simulink model "AutomaticParking_Parallel_UtilityTruck"  (Simulink 10.2)
settings: Solver=ode45  StartTime=0  StopTime=60  FixedStep=0.002  RelTol=1e-3  AbsTol=1e-6
libraries: robotlib x11, Solver_SF x1, simulink x1
(part 1 of 3)
settings Model: Creator=pmather  LastModifiedBy=DwigHT  ExtModeTrigMode=oneshot  ExtModeArmWhenConnect=off
settings OptimizationCC: BlockReduction=off  BooleanDataType=off  InitFltsAndDblsToZero=on  LifeSpan=auto
settings DebuggingCC: SaveWithParameterizedLinksMsg=none  SignalResolutionControl=TryResolveAllWithWarning  MultiTaskDSMMsg=warning  MultiTaskCondExecSysMsg=none  FcnCallInpInsideContextMsg=error  SFUnexpectedBacktrackingDiag=error  SFNoUnconditionalDefaultTransitionDiag=error  SFExecutionAtInitializationDiag=warning
settings HardwareCC: TargetUnknown=on
settings SFSimCC: SimUseLocalCustomCode=on
settings RTWCC: TemplateMakefile=grt_vc.tmf  RTWUseLocalCustomCode=on
settings CodeAppCC: StateflowObjectComments=off
settings ConfigComp: CovExternalEMLEnable=on

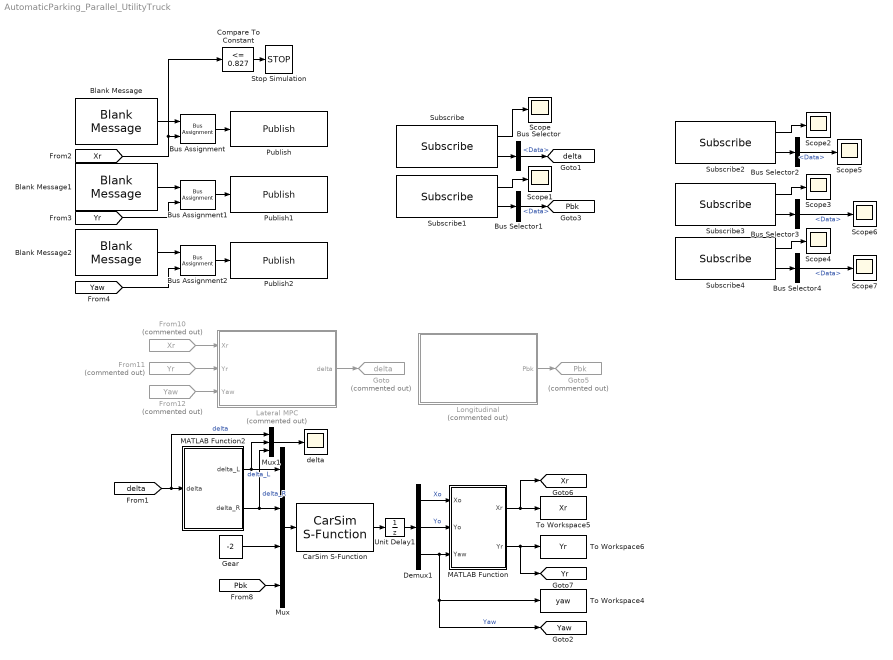
== system AutomaticParking_Parallel_UtilityTruck ==
  Blank Message : robotlib/Blank Message  messageClass=Message  entityType=std_msgs/Float64  messageType=std_msgs/Float64  SampleTime=inf  legacyBusStruct=off
  Blank Message1 : robotlib/Blank Message  messageClass=Message  entityType=std_msgs/Float64  messageType=std_msgs/Float64  SampleTime=inf  legacyBusStruct=off
  Blank Message2 : robotlib/Blank Message  messageClass=Message  entityType=std_msgs/Float64  messageType=std_msgs/Float64  SampleTime=inf  legacyBusStruct=off
  Bus Assignment : BusAssignment  AssignedSignals=Data
  Bus Assignment1 : BusAssignment  AssignedSignals=Data
  Bus Assignment2 : BusAssignment  AssignedSignals=Data
  Bus Selector{,1..4} (5 alike) : BusSelector  OutputSignals=Data
  CarSim S-Function : Solver_SF/CarSim S-Function  Priority=1  VehicleCode=i_s  SIMFILE=simfile
  Compare To Constant : simulink/Logic and Bit Operations/Compare To Constant  relop=<=  const=0.827  OutDataTypeStr=boolean
  Demux1 : Demux  Outputs=3
  From10 : From  Commented=on  GotoTag=Xr  TagVisibility=global
  From11 : From  Commented=on  GotoTag=Yr  TagVisibility=global
  From12 : From  Commented=on  GotoTag=Yaw  TagVisibility=global
  Gear : Constant  Value=-2
  Goto : Goto  Commented=on  GotoTag=delta  TagVisibility=global
  Goto5 : Goto  Commented=on  GotoTag=Pbk  TagVisibility=global
  Lateral MPC : Subsystem  Commented=on
  Longitudinal : Subsystem  Commented=on
  MATLAB Function : MATLAB Function  TreatAsAtomicUnit=on
  MATLAB Function2 : MATLAB Function  TreatAsAtomicUnit=on
  Mux : Mux
  Mux1 : Mux  Inputs=3
  Publish : robotlib/Publish  topicSource=Specify your own  topic=/Xr  messageType=std_msgs/Float64  legacyBusStruct=off  messageQueueLength=1
  Publish1 : robotlib/Publish  topicSource=Specify your own  topic=/Yr  messageType=std_msgs/Float64  legacyBusStruct=off  messageQueueLength=1
  Publish2 : robotlib/Publish  topicSource=Specify your own  topic=/Yaw  messageType=std_msgs/Float64  legacyBusStruct=off  messageQueueLength=1
  Scope{,1..7} (8 alike) : Scope
  Stop Simulation : Stop
  Subscribe : robotlib/Subscribe  topicSource=Specify your own  topic=/delta  messageType=std_msgs/Float64  SampleTime=-1  legacyBusStruct=off  messageQueueLength=1
  Subscribe1 : robotlib/Subscribe  topicSource=Specify your own  topic=/Pbk  messageType=std_msgs/Float64  SampleTime=-1  legacyBusStruct=off  messageQueueLength=1
  Subscribe2 : robotlib/Subscribe  topicSource=Specify your own  topic=/delta_t  messageType=std_msgs/Float64  SampleTime=-1  legacyBusStruct=off  messageQueueLength=1
  Subscribe3 : robotlib/Subscribe  topicSource=Specify your own  topic=/fval  messageType=std_msgs/Float64  SampleTime=-1  legacyBusStruct=off  messageQueueLength=1
  Subscribe4 : robotlib/Subscribe  topicSource=Specify your own  topic=/exitflag  messageType=std_msgs/Float64  SampleTime=-1  legacyBusStruct=off  messageQueueLength=1
  To Workspace4 : ToWorkspace  VariableName=yaw  SaveFormat=Timeseries  SampleTime=-1
  To Workspace5 : ToWorkspace  VariableName=Xr  SaveFormat=Timeseries  SampleTime=-1
  To Workspace6 : ToWorkspace  VariableName=Yr  SaveFormat=Timeseries  SampleTime=-1
  Unit Delay1 : UnitDelay  InitialCondition=[9.432 1.1 0]  SampleTime=-1  HasFrameUpgradeWarning=on
  delta : Scope
  tag scope: Pbk=global, Xr=global, Yaw=global, Yr=global, delta=global
  wires:
  Mux/1 -> CarSim S-Function/1
  CarSim S-Function/1 -> Unit Delay1/1
  Demux1/1 -> MATLAB Function/1(Xo)  "Xo"
  Demux1/2 -> MATLAB Function/2(Yo)  "Yo"
  Demux1/3 -> MATLAB Function/3(Yaw), To Workspace4/1, [Yaw]  "Yaw"
  Gear/1 -> Mux/3
  MATLAB Function2/1(delta_L) -> Mux1/2, Mux/1  "delta_L"
  MATLAB Function2/2(delta_R) -> Mux1/3, Mux/2  "delta_R"
  [delta] -> Mux1/1, MATLAB Function2/1(delta)  "delta"
  Mux1/1 -> delta/1
  MATLAB Function/1(Xr) -> [Xr], To Workspace5/1
  [Pbk] -> Mux/4
  MATLAB Function/2(Yr) -> To Workspace6/1, [Yr]
  From11/1 -> Lateral MPC/2(Yr)
  From10/1 -> Lateral MPC/1(Xr)
  From12/1 -> Lateral MPC/3(Yaw)
  Lateral MPC/1(delta) -> Goto/1
  Longitudinal/1(Pbk) -> Goto5/1
  Unit Delay1/1 -> Demux1/1
  Bus Selector1/1 -> [Pbk]  "<Data>"
  Bus Selector/1 -> [delta]  "<Data>"
  [Yaw] -> Bus Assignment2/2
  [Xr] -> Compare To Constant/1, Bus Assignment/2
  [Yr] -> Bus Assignment1/2
  Blank Message/1 -> Bus Assignment/1
  Bus Assignment/1 -> Publish/1
  Bus Assignment1/1 -> Publish1/1
  Blank Message1/1 -> Bus Assignment1/1
  Blank Message2/1 -> Bus Assignment2/1
  Bus Assignment2/1 -> Publish2/1
  Subscribe/2 -> Bus Selector/1
  Subscribe1/2 -> Bus Selector1/1
  Subscribe/1 -> Scope/1
  Subscribe1/1 -> Scope1/1
  Subscribe2/1 -> Scope2/1
  Subscribe2/2 -> Bus Selector2/1
  Bus Selector2/1 -> Scope5/1  "<Data>"
  Bus Selector3/1 -> Scope6/1  "<Data>"
  Subscribe3/2 -> Bus Selector3/1
  Subscribe3/1 -> Scope3/1
  Subscribe4/1 -> Scope4/1
  Subscribe4/2 -> Bus Selector4/1
  Bus Selector4/1 -> Scope7/1  "<Data>"
  Compare To Constant/1 -> Stop Simulation/1

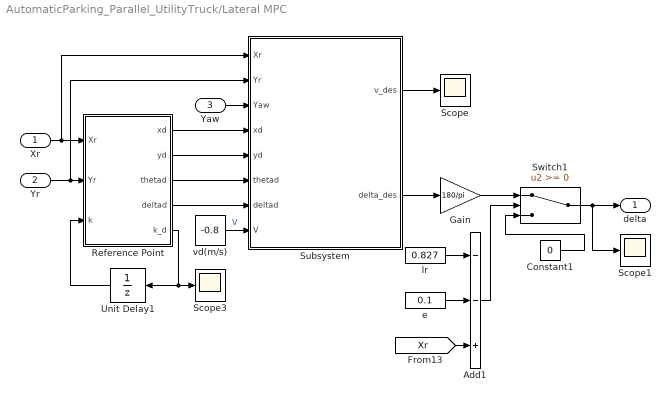
== system AutomaticParking_Parallel_UtilityTruck/Lateral MPC ==
  Xr : Inport
  Yr : Inport  Port=2
  Yaw : Inport  Port=3
  Add1 : Sum  Inputs=--+
  Constant1 : Constant  Value=0
  Gain : Gain  Gain=180/pi
  Reference Point : MATLAB Function  TreatAsAtomicUnit=on
  Scope : Scope
  Scope1 : Scope
  Scope3 : Scope
  Subsystem : Subsystem
  Switch1 : Switch
  Unit Delay1 : UnitDelay  InitialCondition=1  SampleTime=-1  HasFrameUpgradeWarning=on
  e : Constant  Value=0.1
  lr : Constant  Value=0.827
  vd(m/s) : Constant  Value=-0.8
  delta : Outport  VectorParamsAs1DForOutWhenUnconnected=off
  wires:
  Reference Point/2(yd) -> Subsystem/5(yd)
  vd(m/s)/1 -> Subsystem/8(V)  "V"
  Reference Point/4(deltad) -> Subsystem/7(deltad)
  Reference Point/3(thetad) -> Subsystem/6(thetad)
  Unit Delay1/1 -> Reference Point/3(k)
  Reference Point/1(xd) -> Subsystem/4(xd)
  Reference Point/5(k_d) -> Scope3/1, Unit Delay1/1
  Switch1/1 -> Scope1/1, delta/1
  Gain/1 -> Switch1/1
  Xr/1 -> Subsystem/1(Xr), Reference Point/1(Xr)
  Yr/1 -> Subsystem/2(Yr), Reference Point/2(Yr)
  Yaw/1 -> Subsystem/3(Yaw)
  Subsystem/1(v_des) -> Scope/1
  Subsystem/2(delta_des) -> Gain/1
  e/1 -> Add1/2
  lr/1 -> Add1/1
  Constant1/1 -> Switch1/3
  Add1/1 -> Switch1/2
  [Xr] -> Add1/3

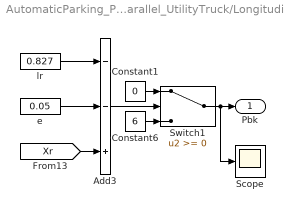
== system AutomaticParking_Parallel_UtilityTruck/Longitudinal ==
  Add3 : Sum  Inputs=--+
  Constant1 : Constant  Value=0
  Constant6 : Constant  Value=6
  Scope : Scope
  Switch1 : Switch
  e : Constant  Value=0.05
  lr : Constant  Value=0.827
  Pbk : Outport  VectorParamsAs1DForOutWhenUnconnected=off
  wires:
  Constant6/1 -> Switch1/3
  Add3/1 -> Switch1/2
  [Xr] -> Add3/3
  e/1 -> Add3/2
  lr/1 -> Add3/1
  Constant1/1 -> Switch1/1
  Switch1/1 -> Scope/1, Pbk/1

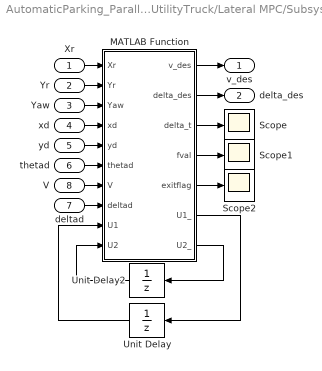
== system AutomaticParking_Parallel_UtilityTruck/Lateral MPC/Subsystem ==
  Xr : Inport
  Yr : Inport  Port=2
  Yaw : Inport  Port=3
  xd : Inport  Port=4
  yd : Inport  Port=5
  thetad : Inport  Port=6
  deltad : Inport  Port=7
  V : Inport  Port=8
  MATLAB Function : MATLAB Function  TreatAsAtomicUnit=on
  Scope : Scope
  Scope1 : Scope
  Scope2 : Scope
  Unit Delay : UnitDelay  SampleTime=-1  HasFrameUpgradeWarning=on
  Unit Delay2 : UnitDelay  SampleTime=-1  HasFrameUpgradeWarning=on
  v_des : Outport
  delta_des : Outport  Port=2
  wires:
  Unit Delay/1 -> MATLAB Function/9(U1)
  MATLAB Function/7(U2_) -> Unit Delay2/1
  Unit Delay2/1 -> MATLAB Function/10(U2)
  Yr/1 -> MATLAB Function/2(Yr)
  MATLAB Function/3(delta_t) -> Scope/1
  yd/1 -> MATLAB Function/5(yd)
  MATLAB Function/6(U1_) -> Unit Delay/1
  MATLAB Function/5(exitflag) -> Scope2/1
  xd/1 -> MATLAB Function/4(xd)
  V/1 -> MATLAB Function/7(V)
  MATLAB Function/1(v_des) -> v_des/1
  Xr/1 -> MATLAB Function/1(Xr)
  Yaw/1 -> MATLAB Function/3(Yaw)
  thetad/1 -> MATLAB Function/6(thetad)
  MATLAB Function/4(fval) -> Scope1/1
  MATLAB Function/2(delta_des) -> delta_des/1
  deltad/1 -> MATLAB Function/8(deltad)

== matlab function MATLAB Function ==
  data: Xo input double; Xr output double; Yo input double; Yaw input double; Yr output double
function [Xr,Yr] = fcn(Xo,Yo,Yaw)
l=1.923;%轴距
Xr=Xo-l*cos(Yaw/180*pi);
Yr=Yo-l*sin(Yaw/180*pi);
